simulink model "Motor_control_S32K_Final"  (R2018b)
settings: Solver=FixedStepDiscrete  StartTime=0.0  StopTime=2  RelTol=1e-3
InitFcn:
  | mbd_s32k14_consistency_checks(bdroot(gcs));
model workspace (MAT data in the model file):
  C_LST = 0.0001
  Nmax = 10000
  PP = 2
  S_LST = 0.001
undefined symbols (not defined in the file): LQFP
libraries: mbd_s32k14_ec_toolbox x13, ammclib_bam_s32k14x x9, simulink x2
Description:
  | This model is used to verify in simulation environment the correct generation
  | of PWM duty cycle commands.
  | 
  | For PWM commands generation, a special NXP library block is used.
  | The GMCLIB_SvmStd function for calculating duty-cycle ratios is widely-used
  | in the modern electric drive. This, function calculates appropriate duty-cycle
  | ratios, which are needed for generating the given stator reference voltage
  | vector using a special Space Vector Modulation technique.
  | 
  | The basic principle of Space Vector Modulation is to approximate the
  | reference stator voltage vector with an appropriate combination
  | of the switching patterns composed of basic space vectors.
  | 
  | For details, please refer to AMMCLIB User Guide, GMCLIB_SvmStd chapter.
  | 
  | For simplicity, a V/f scalar control is simulated to check the correctness of the
  | model prior of testion on the real hardware.
  | 
  | Scope of this model:
  | - demonstrate how to generate the reference signals needed for control
  | - introduce the AMMCLIB special functions for FOC transformations
  | - verify the SVM prior to testing on real hardware
settings Model: Creator=B21307  LastModifiedBy=Arjun
settings DataIOCC: ExternalInput=off  InitialState=off  SaveOutput=off  SignalLogging=off  SaveTime=off
settings OptimizationCC: DefaultParameterBehavior=Inlined  LifeSpan=inf
settings DebuggingCC: InheritedTsInSrcMsg=none  SingleTaskRateTransMsg=error  ParameterPrecisionLossMsg=none  ParameterTunabilityLossMsg=error  UnconnectedInputMsg=error  UnconnectedOutputMsg=error  UnconnectedLineMsg=error  UnknownTsInhSupMsg=error  SFExecutionAtInitializationDiag=none
settings HardwareCC: ProdBitPerPointer=32  ProdBitPerSizeT=32  ProdBitPerPtrDiffT=32  ProdLargestAtomicInteger=Long  ProdLargestAtomicFloat=Double  ProdWordSize=32  ProdHWDeviceType=ARM Compatible->ARM Cortex
settings SFSimCC: SimUseLocalCustomCode=off  MATLABDynamicMemAlloc=off
settings RTWCC: SystemTargetFile=mbd_s32k14.tlc  MakeCommand=mbd_s32k14_make_rtw COPY_MDLREF_INCLUDES=0  TemplateMakefile=mbd_s32k14.tmf  Description=Model Based Design Toolbox S32K14x Code Generation Target  RTWUseLocalCustomCode=off  IncludeHyperlinkInReport=on
settings CodeAppCC: ForceParamTrailComments=on  IgnoreCustomStorageClasses=off  OperatorAnnotations=on  SimulinkDataObjDesc=on  SFDataObjDesc=on  InsertBlockDesc=on  StateflowObjectComments=on
settings STFCustomTargetCC: TargetLangStandard=C99 (ISO)  MultiwordLength=256  CombineOutputUpdateFcns=on  ERTCustomFileBanners=on  SupportContinuousTime=off  SupportNonInlinedSFcns=off  RemoveResetFunc=on  MATLABClassNameForMDSCustomization=Simulink.SoftwareTarget.ERTCustomization  SystemTargetFile=mbd_s32k14.tlc
settings ERTTargetCC: TargetLangStandard=C99 (ISO)  ParMdlRefBuildCompliant=off  CompOptLevelCompliant=off  ConcurrentExecutionCompliant=off  ModelStepFunctionPrototypeControlCompliant=off  CPPClassGenCompliant=off  UseToolchainInfoCompliant=off  InlinedParameterPlacement=NonHierarchical  ERTCustomFileTemplate=example_file_process.tlc

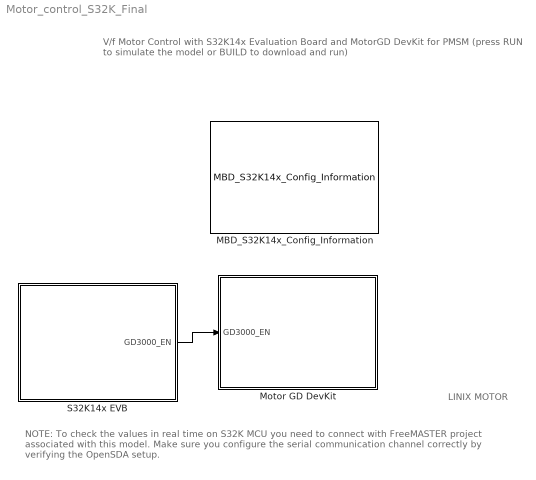
== system Motor_control_S32K_Final ==
  note: LINIX MOTOR
  note: V/f Motor Control
      | with S32K14x Evaluation Board and MotorGD DevKit for PMSM
      | (press RUN to simulate the model or BUILD to download and run)
  note: NOTE: To check the values in real time on S32K MCU you need to connect with FreeMASTER project associated with this model. Make sure you configure the serial communication channel correctly by verifying the OpenSDA setup.
  MBD_S32K14x_Config_Information : mbd_s32k14_ec_toolbox/MBD_S32K14x_Config_Information  Priority=1  disp_str=|  config_params=[]  mcu_target_name=S32K144  mcu_target_package=100-LQFP  mcu_target_sram_size=64KB  mcu_system_clock_freq=80  mcu_xtal_freq=External 8  mcu_steptick_timer=LPIT Channel 0  mcu_steptick_prio=15  ds_import_enable=on  target_compiler=GCC  target_memory=FLASH  gcc_target_compile_opts=-mcpu=cortex-m4 -mthumb -mfloat-abi=hard -mfpu=fpv4-sp-d16 -O1 -g -gstrict-dwarf  gcc_target_assemble_opts=-mcpu=cortex-m4 -mthumb -mfloat-abi=hard -mfpu=fpv4-sp-d16 -g  gcc_target_link_opts=-mcpu=cortex-m4 -mthumb -mfloat-abi=hard -mfpu=fpv4-sp-d16  gcc_target_default_lcf=on  gcc_target_user_lcf=S32K148_256_flash.ld  ghs_target_compile_opts=-cpu=cortexm4f -thumb -fpu=vfpv4_d16 -fsingle -Ogeneral -Wundef -Wimplicit-int -Wshadow -Wtrigraphs --no_commons --gnu_asm -gnu99 -gdwarf-2 -G  ghs_target_assemble_opts=-cpu=cortexm4f -fpu=vfpv4_d16  ghs_target_link_opts=-cpu=cortexm4f -thumb -fpu=vfpv4_d16  ghs_target_default_lcf=on  ghs_target_user_lcf=S32K148_256_flash.ld  iar_target_compile_opts=--cpu=Cortex-M4F --thumb --fpu=VFPv4_sp -Ol -e --debug --dlib_config normal  iar_target_assemble_opts=--cpu Cortex-M4F --thumb --fpu VFPv4_sp  iar_target_link_opts=--no_exceptions --vfe --inline  iar_target_default_lcf=on  iar_target_user_lcf=S32K148_256_flash.icf  pil_download_enable=off  rbl_download_enable=on  rbl_start_delay=5000  rbl_download_interface=OpenSDA  rbl_restart_request=off  rbl_com_port=Custom  rbl_com_port_custom=COM1  pil_download_rate=57600  pil_opensda_drive=Custom  pil_opensda_drive_custom=E  FTM_PWM_PcrCheckEnDis=on  FTM_Input_Edge_Inputs_PcrCheckEnDis=on  FTM_Dual_Edge_Inputs_PcrCheckEnDis=on  FTM_Quadrature_Inputs_PcrCheckEnDis=on  LPTMR_PcrCheckEnDis=on  PIT_PcrCheckEnDis=on  RTC_PcrCheckEnDis=on  FlexCAN_PcrCheckEnDis=on  FlexIO_PcrCheckEnDis=on  LPI2C_PcrCheckEnDis=on  LPSPI_PcrCheckEnDis=on  LPUART_PcrCheckEnDis=on  CMP_PcrCheckEnDis=on  GPIO_OutputPcrCheckEnDis=on  GPIO_InputPcrCheckEnDis=on  SBC_PcrCheckEnDis=on  AMMCLIB_PcrCheckEnDis=on  FM_PcrCheckEnDis=on  Profile_PcrCheckEnDis=on  ConfigParams_PcrCheckEnDis=on  ModelRef_PcrCheckEnDis=on  PDB0_PcrCheckEnDis=on  CSEc_PcrCheckEnDis=on  eDMA_PcrCheckEnDis=on  ADC_PcrCheckEnDis=on
      | Target : S32K144-64KB_SRAM
      | Package : 100-pin
      | System clock : 80 MHz
      | XTAL clock : External 8 MHz
      | Compiler : GCC
      | Target Type : FLASH
      | Download Code after build : (OpenSDA: D)
      | Step Tick Interrupt Priority : 15
  Motor GD DevKit : Subsystem
      mask Display: image('.\img\MotorGD.PNG');
  S32K14x EVB : Subsystem
      mask Display: image('.\img\S32K.PNG');
  wires:
  S32K14x EVB/1(GD3000_EN) -> Motor GD DevKit/1(GD3000_EN)

== system Motor_control_S32K_Final/Motor GD DevKit ==
  note: MotorGD DevKit Configuration
      |
      | PWM Commands are transformed in 3-phase Sinusoidal Voltages with Vdc amplitude
      | Enable the MC34GD3000 pre-driver to allow voltage generation on motor phases
  GD3000_EN : Inport
  GD3000_EN_IO : mbd_s32k14_ec_toolbox/GPIO Blocks/Digital_Output  gpio_pin=PTA2: [PTA2 | Port A I/O]  drive_strength=High
  GD3000_RST_IO : mbd_s32k14_ec_toolbox/GPIO Blocks/Digital_Output  gpio_pin=PTA3: [PTA3 | Port A I/O]  drive_strength=High
  ON : Constant  OutDataTypeStr=boolean
  wires:
  ON/1 -> GD3000_RST_IO/1
  GD3000_EN/1 -> GD3000_EN_IO/1

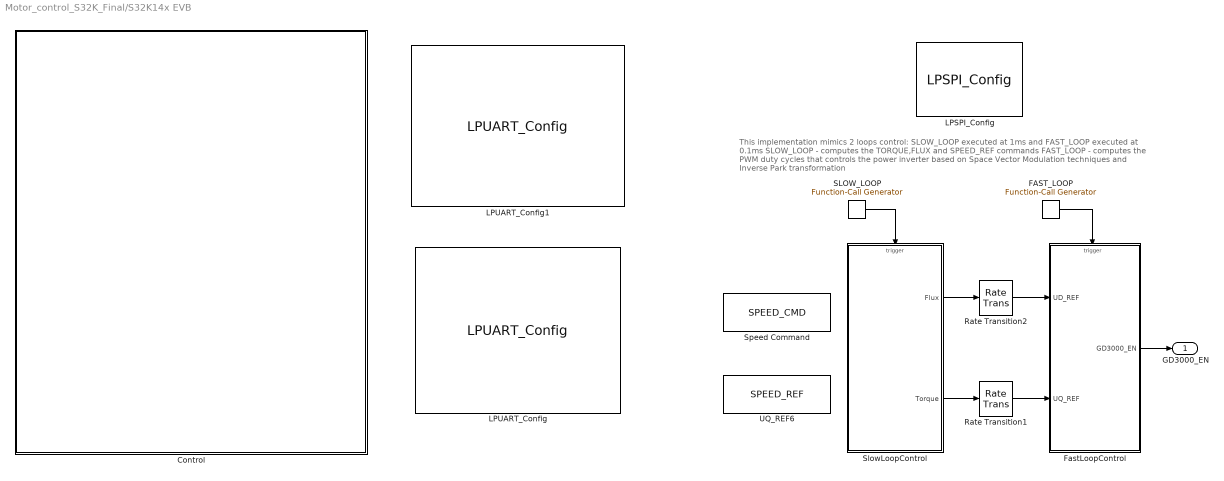
== system Motor_control_S32K_Final/S32K14x EVB ==
  note: This implementation mimics 2 loops control: SLOW_LOOP executed at 1ms and FAST_LOOP executed at 0.1ms
      | SLOW_LOOP - computes the TORQUE,FLUX and SPEED_REF  commands
      | FAST_LOOP  - computes the PWM duty cycles that controls the power inverter based on Space Vector Modulation
      |                          techniques and Inverse Park transformation
  "Control " : Subsystem
  FAST_LOOP : simulink/Ports & Subsystems/Function-Call Generator  sample_time=C_LST  numberOfIterations=1
  FastLoopControl : Subsystem
      settings: RTWFcnNameOpts=Use subsystem name
  "LPSPI_Config " : mbd_s32k14_ec_toolbox/Communication Blocks/SPI Blocks/LPSPI_Config   InstanceNumber=0  Role=Master  BaudRate=1000000  ShowAdvanced=on  sin=PTB3: [LPSPI0_SIN | LPSPI Serial Data Input]  sout=PTB4: [LPSPI0_SOUT | LPSPI Serial Data Output]  sck=PTB2: [LPSPI0_SCK | LPSPI Serial Clock I/O]  pcs0=PTB0: [LPSPI0_PCS0 | Peripheral Chip Select 0]  pcs1=PTB5: [LPSPI0_PCS1 | Peripheral Chip Select 1]  pcs2=PTE6: [LPSPI0_PCS2 | Peripheral Chip Select 2]  pcs3=PTA15: [LPSPI0_PCS3 | Peripheral Chip Select 3]  CPHA=1  CPOL=0  BitOrder=MSB first  TransferSize=8  WhichPCS=1  PCSPol=ActiveLow  ContinuousTransfer=off
  LPUART_Config : mbd_s32k14_ec_toolbox/Communication Blocks/UART Blocks/LPUART_Config  Priority=1  instance=1  baudrate=115200  databits=8  parity=None  sbns=1  bothedge=rising edge  rxinv=off  txinv=off  show_adv_opts=on  brk13=10 - 13 bit times  lbkde=10 - 13 bit times  rx=PTC6: [LPUART1_RX | Receive]  tx=PTC7: [LPUART1_TX | Transmit]  cts=PTA6: [LPUART1_CTS | Clear To Send (bar)]  rts=PTA7: [LPUART1_RTS | Request To Send]
  LPUART_Config1 : mbd_s32k14_ec_toolbox/Communication Blocks/UART Blocks/LPUART_Config  Priority=2  instance=2  baudrate=115200  databits=8  parity=None  sbns=1  bothedge=rising edge  rxinv=off  txinv=off  show_adv_opts=off  brk13=10 - 13 bit times  lbkde=10 - 13 bit times  rx=PTD6: [LPUART2_RX | Receive]  tx=PTD7: [LPUART2_TX | Transmit]  cts=PTD11: [LPUART2_CTS | Clear To Send (bar)]  rts=PTD12: [LPUART2_RTS | Request To Send]
  Rate Transition1 : RateTransition  OutPortSampleTime=C_LST
  Rate Transition2 : RateTransition  OutPortSampleTime=C_LST
  SLOW_LOOP : simulink/Ports & Subsystems/Function-Call Generator  sample_time=S_LST  numberOfIterations=1
  SlowLoopControl : Subsystem
      settings: RTWFcnNameOpts=Use subsystem name
  Speed Command : DataStoreMemory  DataStoreName=SPEED_CMD  ReadBeforeWriteMsg=warning  WriteAfterWriteMsg=warning  WriteAfterReadMsg=warning  ShowAdditionalParam=off  OutMin=-100  OutMax=200  OutDataTypeStr=single
  UQ_REF6 : DataStoreMemory  DataStoreName=SPEED_REF  ReadBeforeWriteMsg=warning  WriteAfterWriteMsg=warning  WriteAfterReadMsg=warning  ShowAdditionalParam=off  OutDataTypeStr=single
  GD3000_EN : Outport
  wires:
  SLOW_LOOP/1 -> SlowLoopControl/Trigger
  Rate Transition2/1 -> FastLoopControl/1(UD_REF)
  Rate Transition1/1 -> FastLoopControl/2(UQ_REF)
  SlowLoopControl/1(Flux) -> Rate Transition2/1
  SlowLoopControl/2(Torque) -> Rate Transition1/1
  FAST_LOOP/1 -> FastLoopControl/Trigger
  FastLoopControl/1(GD3000_EN) -> GD3000_EN/1

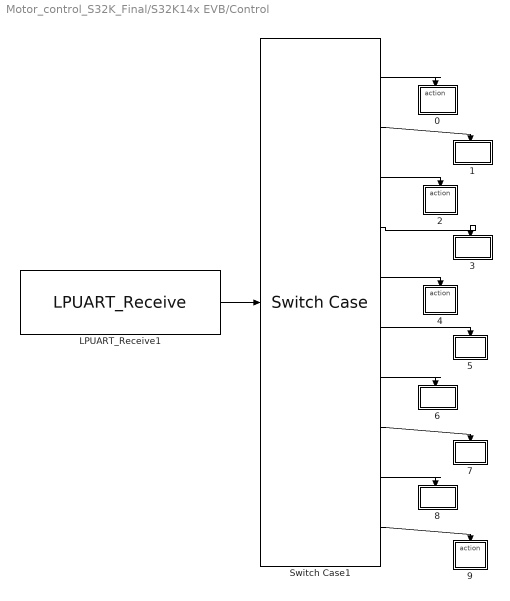
== system Motor_control_S32K_Final/S32K14x EVB/Control  ==
  0 : Subsystem  TreatAsAtomicUnit=on
  1 : Subsystem  TreatAsAtomicUnit=on
  2 : Subsystem  TreatAsAtomicUnit=on
  "3 " : Subsystem  TreatAsAtomicUnit=on
  "4 " : Subsystem  TreatAsAtomicUnit=on
  5 : Subsystem  TreatAsAtomicUnit=on
  6 : Subsystem  TreatAsAtomicUnit=on
  7 : Subsystem  TreatAsAtomicUnit=on
  "8 " : Subsystem  TreatAsAtomicUnit=on
  9 : Subsystem  TreatAsAtomicUnit=on
  LPUART_Receive1 : mbd_s32k14_ec_toolbox/Communication Blocks/UART Blocks/LPUART_Receive  Priority=1  instance=1
  Switch Case1 : SwitchCase  CaseConditions={hex2dec('030'),hex2dec('031'),hex2dec('032'),hex2dec('033'),hex2dec('034'),hex2dec('035'),hex2dec('036'),hex2dec('037'),hex2dec('038'),hex2dec('039')}  ShowDefaultCase=off
  wires:
  Switch Case1/3 -> 2/Action
  Switch Case1/8 -> 7/Action
  Switch Case1/1 -> 0/Action
  LPUART_Receive1/1 -> Switch Case1/1
  Switch Case1/6 -> 5/Action
  Switch Case1/10 -> 9/Action
  Switch Case1/9 -> "8 "/Action
  Switch Case1/5 -> "4 "/Action
  Switch Case1/4 -> "3 "/Action
  Switch Case1/2 -> 1/Action
  Switch Case1/7 -> 6/Action

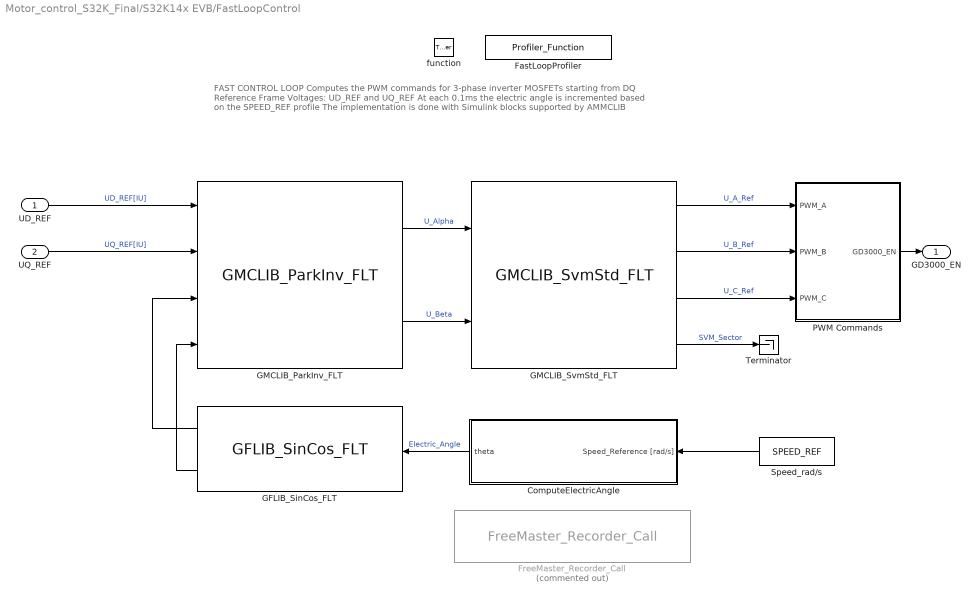
== system Motor_control_S32K_Final/S32K14x EVB/FastLoopControl ==
  note: FAST CONTROL LOOP
      |
      | Computes the PWM commands for 3-phase inverter MOSFETs starting from DQ Reference Frame Voltages: UD_REF and UQ_REF
      | At each 0.1ms the electric angle is incremented based on the SPEED_REF profile
      | The implementation is done with Simulink blocks supported by AMMCLIB
  UD_REF : Inport
  UQ_REF : Inport  Port=2
  function : TriggerPort  TriggerType=function-call  VariantControl=(inherit)
  ComputeElectricAngle : Subsystem  TreatAsAtomicUnit=on
      settings: RTWFcnNameOpts=Use subsystem name
  FastLoopProfiler : mbd_s32k14_ec_toolbox/Utility Blocks/Profiler_Function  profile_indx=0
  FreeMaster_Recorder_Call : mbd_s32k14_ec_toolbox/Utility Blocks/FreeMaster_Recorder_Call  Commented=on
  GFLIB_SinCos_FLT : ammclib_bam_s32k14x/GFLIB/bam_flt/GFLIB_SinCos_FLT
  GMCLIB_ParkInv_FLT : ammclib_bam_s32k14x/GMCLIB/bam_flt/GMCLIB_ParkInv_FLT
  GMCLIB_SvmStd_FLT : ammclib_bam_s32k14x/GMCLIB/bam_flt/GMCLIB_SvmStd_FLT
  PWM Commands : Subsystem
  Speed_rad/s : DataStoreRead  DataStoreName=SPEED_REF
  Terminator : Terminator
  GD3000_EN : Outport
  wires:
  GFLIB_SinCos_FLT/2 -> GMCLIB_ParkInv_FLT/4
  GMCLIB_ParkInv_FLT/1 -> GMCLIB_SvmStd_FLT/1  "U_Alpha"
  GMCLIB_ParkInv_FLT/2 -> GMCLIB_SvmStd_FLT/2  "U_Beta"
  GFLIB_SinCos_FLT/1 -> GMCLIB_ParkInv_FLT/3
  GMCLIB_SvmStd_FLT/2 -> PWM Commands/2(PWM_B)  "U_B_Ref"
  GMCLIB_SvmStd_FLT/3 -> PWM Commands/3(PWM_C)  "U_C_Ref"
  GMCLIB_SvmStd_FLT/4 -> Terminator/1  "SVM_Sector"
  GMCLIB_SvmStd_FLT/1 -> PWM Commands/1(PWM_A)  "U_A_Ref"
  UD_REF/1 -> GMCLIB_ParkInv_FLT/1  "UD_REF[IU]"
  UQ_REF/1 -> GMCLIB_ParkInv_FLT/2  "UQ_REF[IU]"
  ComputeElectricAngle/1(theta) -> GFLIB_SinCos_FLT/1  "Electric_Angle"
  PWM Commands/1(GD3000_EN) -> GD3000_EN/1
  Speed_rad/s/1 -> ComputeElectricAngle/1(Speed_Reference [rad/s])

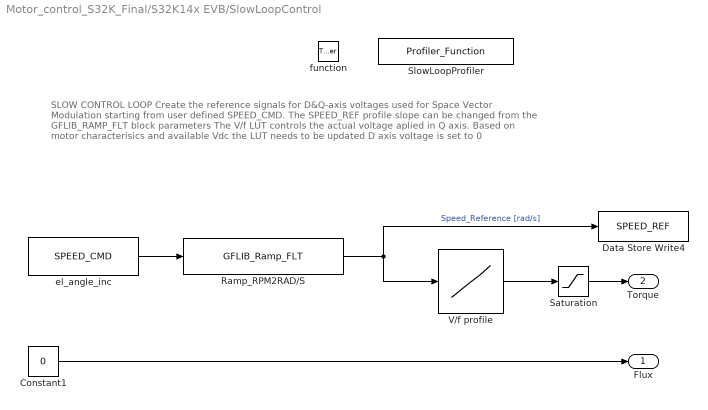
== system Motor_control_S32K_Final/S32K14x EVB/SlowLoopControl ==
  note: SLOW CONTROL LOOP
      |
      | Create the reference signals for D&Q-axis voltages used for Space Vector Modulation starting from user defined SPEED_CMD.
      | The SPEED_REF profile slope can be changed from the GFLIB_RAMP_FLT block parameters
      | The V/f LUT controls the actual voltage aplied in Q axis. Based on motor characterisics and available Vdc the LUT needs to be updated
      | D axis voltage is set to 0
  function : TriggerPort  TriggerType=function-call  VariantControl=(inherit)
  Constant1 : Constant  Value=0  OutDataTypeStr=single  SampleTime=-1
  Data Store Write4 : DataStoreWrite  DataStoreName=SPEED_REF
  Ramp_RPM2RAD/S : ammclib_bam_s32k14x/GFLIB/bam_flt/GFLIB_Ramp_FLT  fltRampUp=0.1  fltRampDown=0.1
  Saturation : Saturate  UpperLimit=0.95  LowerLimit=0
  SlowLoopProfiler : mbd_s32k14_ec_toolbox/Utility Blocks/Profiler_Function  profile_indx=1
  V/f profile : Lookup_n-D  NumberOfTableDimensions=1  BreakpointsForDimension1=[0:20.94:309.4]  Table=[0.20:0.075:0.95]  InternalRulePriority=Speed  RndMeth=Simplest  InputSameDT=on
  el_angle_inc : DataStoreRead  DataStoreName=SPEED_CMD
  Flux : Outport
  Torque : Outport  Port=2
  wires:
  Constant1/1 -> Flux/1
  V/f profile/1 -> Saturation/1
  el_angle_inc/1 -> Ramp_RPM2RAD/S/1
  Saturation/1 -> Torque/1
  Ramp_RPM2RAD/S/1 -> V/f profile/1, Data Store Write4/1  "Speed_Reference [rad/s]"

== system Motor_control_S32K_Final/S32K14x EVB/Control /0 ==
  Action Port : ActionPort  ActionType=case
  Constant : Constant  Value=0  OutDataTypeStr=single
  Data Store Write : DataStoreWrite  DataStoreName=SPEED_CMD
  wires:
  Constant/1 -> Data Store Write/1

== system Motor_control_S32K_Final/S32K14x EVB/Control /1 ==
  Action Port : ActionPort  ActionType=case
  Constant : Constant  Value=100  OutDataTypeStr=single
  Data Store Write : DataStoreWrite  DataStoreName=SPEED_CMD
  wires:
  Constant/1 -> Data Store Write/1

== system Motor_control_S32K_Final/S32K14x EVB/Control /2 ==
  Action Port : ActionPort  ActionType=case
  Constant : Constant  Value=200  OutDataTypeStr=single
  Data Store Write : DataStoreWrite  DataStoreName=SPEED_CMD
  wires:
  Constant/1 -> Data Store Write/1

== system Motor_control_S32K_Final/S32K14x EVB/Control /3  ==
  Action Port : ActionPort  ActionType=case
  Constant : Constant  Value=300  OutDataTypeStr=single
  Data Store Write : DataStoreWrite  DataStoreName=SPEED_CMD
  wires:
  Constant/1 -> Data Store Write/1

== system Motor_control_S32K_Final/S32K14x EVB/Control /4  ==
  Action Port : ActionPort  ActionType=case
  Constant : Constant  Value=400  OutDataTypeStr=single
  Data Store Write : DataStoreWrite  DataStoreName=SPEED_CMD
  wires:
  Constant/1 -> Data Store Write/1

== system Motor_control_S32K_Final/S32K14x EVB/Control /5 ==
  Action Port : ActionPort  ActionType=case
  Constant : Constant  Value=500  OutDataTypeStr=single
  Data Store Write : DataStoreWrite  DataStoreName=SPEED_CMD
  wires:
  Constant/1 -> Data Store Write/1

== system Motor_control_S32K_Final/S32K14x EVB/Control /6 ==
  Action Port : ActionPort  ActionType=case
  Constant : Constant  Value=600  OutDataTypeStr=single
  Data Store Write : DataStoreWrite  DataStoreName=SPEED_CMD
  wires:
  Constant/1 -> Data Store Write/1

== system Motor_control_S32K_Final/S32K14x EVB/Control /7 ==
  Action Port : ActionPort  ActionType=case
  Constant : Constant  Value=800  OutDataTypeStr=single
  Data Store Write1 : DataStoreWrite  DataStoreName=SPEED_REF
  wires:
  Constant/1 -> Data Store Write1/1

== system Motor_control_S32K_Final/S32K14x EVB/Control /8  ==
  Action Port : ActionPort  ActionType=case
  Constant : Constant  Value=2100  OutDataTypeStr=single
  Data Store Write : DataStoreWrite  DataStoreName=SPEED_REF
  wires:
  Constant/1 -> Data Store Write/1

== system Motor_control_S32K_Final/S32K14x EVB/Control /9 ==
  Action Port : ActionPort  ActionType=case
  Constant : Constant  Value=4000  OutDataTypeStr=single
  Data Store Write1 : DataStoreWrite  DataStoreName=SPEED_REF
  wires:
  Constant/1 -> Data Store Write1/1

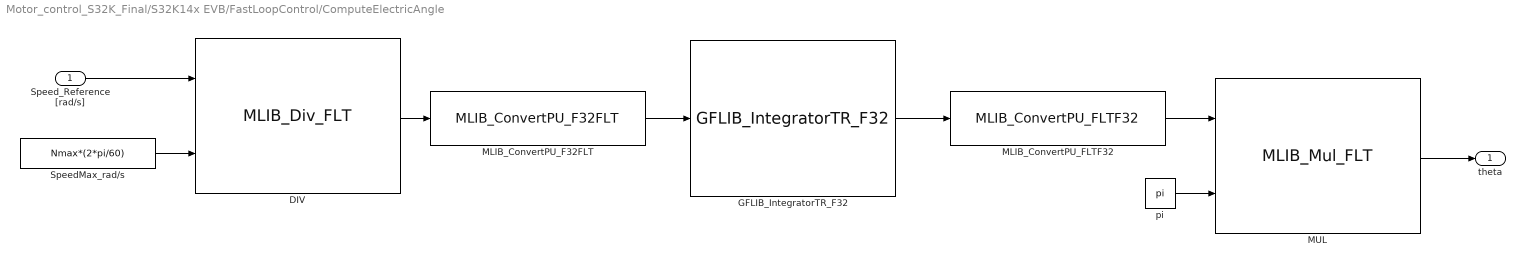
== system Motor_control_S32K_Final/S32K14x EVB/FastLoopControl/ComputeElectricAngle ==
  Speed_Reference [rad/s] : Inport
  DIV : ammclib_bam_s32k14x/MLIB/bam_flt/MLIB_Div_FLT
  GFLIB_IntegratorTR_F32 : ammclib_bam_s32k14x/GFLIB/bam_f32/GFLIB_IntegratorTR_F32  f32C1=(2*pi/60)*PP*Nmax*(C_LST/2/pi)*(2^31)  u16NShift=0
  MLIB_ConvertPU_F32FLT : ammclib_bam_s32k14x/MLIB/bam_f32/MLIB_ConvertPU_F32FLT
  MLIB_ConvertPU_FLTF32 : ammclib_bam_s32k14x/MLIB/bam_flt/MLIB_ConvertPU_FLTF32
  MUL : ammclib_bam_s32k14x/MLIB/bam_flt/MLIB_Mul_FLT
  SpeedMax_rad/s : Constant  Value=Nmax*(2*pi/60)  OutDataTypeStr=Inherit: Inherit via back propagation
  pi : Constant  Value=pi  OutDataTypeStr=Inherit: Inherit via back propagation
  theta : Outport  OutDataTypeStr=single
  wires:
  pi/1 -> MUL/2
  GFLIB_IntegratorTR_F32/1 -> MLIB_ConvertPU_FLTF32/1
  MLIB_ConvertPU_F32FLT/1 -> GFLIB_IntegratorTR_F32/1
  MLIB_ConvertPU_FLTF32/1 -> MUL/1
  MUL/1 -> theta/1
  Speed_Reference [rad/s]/1 -> DIV/1
  DIV/1 -> MLIB_ConvertPU_F32FLT/1
  SpeedMax_rad/s/1 -> DIV/2

== system Motor_control_S32K_Final/S32K14x EVB/FastLoopControl/PWM Commands ==
  PWM_A : Inport
  PWM_B : Inport  Port=2
  PWM_C : Inport  Port=3
  Control_Logic : Subsystem
  Demux : Demux  Outputs=6
  FTM_PWM_Config : mbd_s32k14_ec_toolbox/Motor Control Blocks/FTM Blocks/FTM_PWM_Config  ftmModule=3  ftmMode=Center-Aligned PWM  ftmSourceClock=80 MHz  chan0En=on  chan0Type=Independent  chan2En=on  chan2Type=Independent  chan4En=on  chan4Type=Independent  chan6En=off  chan6Type=Independent  ftmPwmUnits=Hz  outFrequency=20000  ftmPeriod=4000  ftmPrescaler=Divide by 1  deadtimeUnits=Ticks  deadtimeNs=0  deadtimeTicks=0  deadtimePrescaler=Divide by 1  dutyCycleCh0=0  dutyCycleCh1=0  dutyCycleCh2=0  dutyCycleCh3=0  dutyCycleCh4=0  dutyCycleCh5=0  dutyCycleCh6=0.25  dutyCycleCh7=0.25  dutyCycleSim=off  startAfterInit=off  showAdvOpt=on  pinFtmCh0=PTB8: [FTM3_CH0 | FTM Channel]  pinFtmCh1=PTB9: [FTM3_CH1 | FTM Channel]  pinPolCh0=Active Low  pinPolCh1=Main duplicated  outputLevel0=Low-true pulses  outputLevel1=High-true pulses  pinFtmCh2=PTB10: [FTM3_CH2 | FTM Channel]  pinFtmCh3=PTB11: [FTM3_CH3 | FTM Channel]  pinPolCh2=Active Low  pinPolCh3=Main duplicated  outputLevel2=Low-true pulses  outputLevel3=High-true pulses  pinFtmCh4=PTC10: [FTM3_CH4 | FTM Channel]  pinFtmCh5=PTC11: [FTM3_CH5 | FTM Channel]  pinPolCh4=Active Low  pinPolCh5=Main duplicated  outputLevel4=Low-true pulses  outputLevel5=High-true pulses  pinFtmCh6=PTC12: [FTM3_CH6 | FTM Channel]  pinFtmCh7=None  pinPolCh6=Active Low  pinPolCh7=Main duplicated  outputLevel6=High-true pulses  outputLevel7=High-true pulses  initTrigger=off  chTrigger0=off  chTrigger1=off  chTrigger2=off  chTrigger3=off  chTrigger4=off  chTrigger5=off  chTrigger6=off  chTrigger7=off  mcuTargetUpdate=on  pwmSyncTrg=Software trigger  pwmSyncHwRouting=TRGMUX_FTM7  pwmSyncTrg0=off  pwmSyncTrg1=off  pwmSyncTrg2=off  pwmSyncAutoClear=on  pwmSyncMinLoad=on  pwmSyncMaxLoad=on  pwmSyncInvert=System Clock  pwmSyncOutControl=System Clock  pwmSyncOutMask=System Clock  pwmSyncCounterInitial=System Clock  pwmSyncPoints=Update now  reloadEnable=off  reloadPriority=15  reloadHalfCycle=off  reloadHCR=0  reloadFrequency=0  chnMatch0=off  chnMatch1=off  chnMatch2=off  chnMatch3=off  chnMatch4=off  chnMatch5=off  chnMatch6=off  chnMatch7=off  pwmFaultProtection=off  pwmFaultInterrupt=off  pwmFaultClearing=Fault control disabled  pwmFaultPinState=Safe Value  pwmFaultFilterValue=0  pwmFaultPriority=15  fault_disen_0=off  fault_filter_0=off  fault_polarity_0=Active High  fault_disen_1=off  fault_filter_1=off  fault_polarity_1=Active high  fault_disen_2=off  fault_filter_2=off  fault_polarity_2=Active high  fault_disen_3=off  fault_filter_3=off  fault_polarity_3=Active high  fault_pin_0=None  fault_pin_1=None  fault_pin_2=None  fault_pin_3=None
  Mux : Mux  Inputs=6
  GD3000_EN : Outport
  wires:
  Mux/1 -> Control_Logic/1(PWM)
  Control_Logic/1("PWM ") -> Demux/1
  Control_Logic/2(GD3000_EN) -> GD3000_EN/1
  Demux/2 -> FTM_PWM_Config/2  "PA_LS"
  Demux/1 -> FTM_PWM_Config/1  "PA_HS"
  Demux/3 -> FTM_PWM_Config/3  "PB_HS"
  Demux/4 -> FTM_PWM_Config/4  "PB_LS"
  Demux/5 -> FTM_PWM_Config/5  "PC_HS"
  Demux/6 -> FTM_PWM_Config/6  "PC_LS"
  PWM_A/1 -> Mux/2, Mux/1  "PWM_A"
  PWM_B/1 -> Mux/3, Mux/4  "PWM_B"
  PWM_C/1 -> Mux/6, Mux/5  "PWM_C"

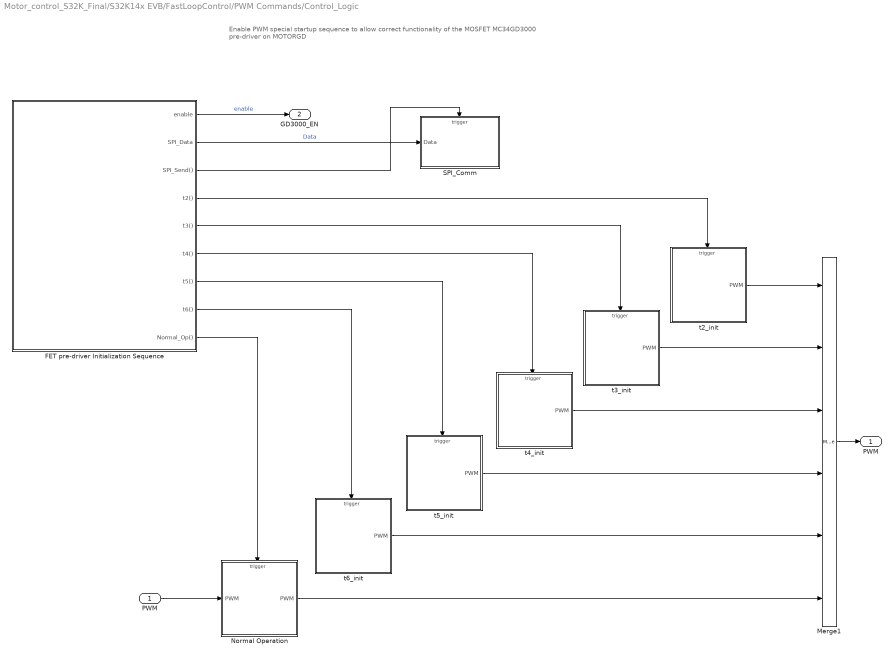
== system Motor_control_S32K_Final/S32K14x EVB/FastLoopControl/PWM Commands/Control_Logic ==
  note: Enable PWM special startup sequence to allow correct functionality of the MOSFET MC34GD3000 pre-driver on MOTORGD
  PWM : Inport
  FET pre-driver Initialization Sequence : Stateflow chart  TreatAsAtomicUnit=on
  Merge1 : Merge  Inputs=6
  Normal Operation : Subsystem  TreatAsAtomicUnit=on
  SPI_Comm : Subsystem
  t2_init : Subsystem  TreatAsAtomicUnit=on
  t3_init : Subsystem  TreatAsAtomicUnit=on
  t4_init : Subsystem  TreatAsAtomicUnit=on
  t5_init : Subsystem  TreatAsAtomicUnit=on
  t6_init : Subsystem  TreatAsAtomicUnit=on
  "PWM " : Outport
  GD3000_EN : Outport  Port=2
  wires:
  FET pre-driver Initialization Sequence/8(t6()) -> t6_init/Trigger
  FET pre-driver Initialization Sequence/7(t5()) -> t5_init/Trigger
  PWM/1 -> Normal Operation/1("PWM ")
  FET pre-driver Initialization Sequence/1(enable) -> GD3000_EN/1  "enable"
  FET pre-driver Initialization Sequence/9(Normal_Op()) -> Normal Operation/Trigger
  FET pre-driver Initialization Sequence/6(t4()) -> t4_init/Trigger
  FET pre-driver Initialization Sequence/5(t3()) -> t3_init/Trigger
  FET pre-driver Initialization Sequence/4(t2()) -> t2_init/Trigger
  Normal Operation/1(PWM) -> Merge1/6
  Merge1/1 -> "PWM "/1
  t2_init/1(PWM) -> Merge1/1
  t3_init/1(PWM) -> Merge1/2
  t4_init/1(PWM) -> Merge1/3
  t5_init/1(PWM) -> Merge1/4
  t6_init/1(PWM) -> Merge1/5
  FET pre-driver Initialization Sequence/2(SPI_Data) -> SPI_Comm/1(Data)  "Data"
  FET pre-driver Initialization Sequence/3(SPI_Send()) -> SPI_Comm/Trigger

== system Motor_control_S32K_Final/S32K14x EVB/FastLoopControl/PWM Commands/Control_Logic/Normal Operation ==
  "PWM " : Inport  OutDataTypeStr=single
  function : TriggerPort  TriggerType=function-call  VariantControl=(inherit)
  PWM : Outport  InitialOutput=0
  wires:
  "PWM "/1 -> PWM/1

== system Motor_control_S32K_Final/S32K14x EVB/FastLoopControl/PWM Commands/Control_Logic/SPI_Comm ==
  Data : Inport
  function : TriggerPort  TriggerType=function-call  VariantControl=(inherit)
  LPSPI_Master_Transfer : mbd_s32k14_ec_toolbox/Communication Blocks/SPI Blocks/LPSPI_Master_Transfer  instance=0  xfermode=Non blocking  timeout=50  spi_upd=on
  Terminator : Terminator
  wires:
  Data/1 -> LPSPI_Master_Transfer/1
  LPSPI_Master_Transfer/1 -> Terminator/1

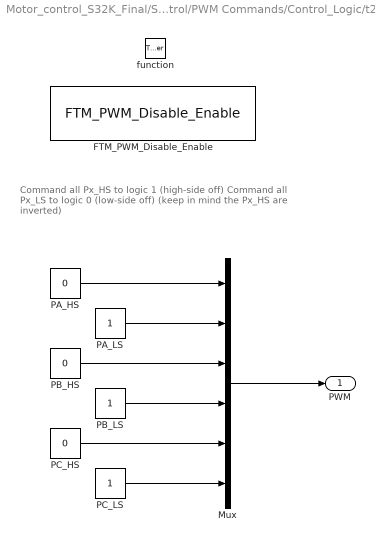
== system Motor_control_S32K_Final/S32K14x EVB/FastLoopControl/PWM Commands/Control_Logic/t2_init ==
  note: Command all Px_HS to logic 1 (high-side off)
      | Command all Px_LS to logic 0 (low-side off)
      | (keep in mind the Px_HS are inverted)
  function : TriggerPort  TriggerType=function-call  VariantControl=(inherit)
  FTM_PWM_Disable_Enable : mbd_s32k14_ec_toolbox/Motor Control Blocks/FTM Blocks/FTM_PWM_Disable_Enable  Priority=1  module=3  action=Enable
  Mux : Mux  Inputs=6
  PA_HS : Constant  Value=0  OutDataTypeStr=single  SampleTime=-1
  PA_LS : Constant  OutDataTypeStr=single  SampleTime=-1
  PB_HS : Constant  Value=0  OutDataTypeStr=single  SampleTime=-1
  PB_LS : Constant  OutDataTypeStr=single  SampleTime=-1
  PC_HS : Constant  Value=0  OutDataTypeStr=single  SampleTime=-1
  PC_LS : Constant  OutDataTypeStr=single  SampleTime=-1
  PWM : Outport  OutDataTypeStr=single  InitialOutput=0
  wires:
  PA_HS/1 -> Mux/1
  Mux/1 -> PWM/1
  PA_LS/1 -> Mux/2
  PB_HS/1 -> Mux/3
  PB_LS/1 -> Mux/4
  PC_HS/1 -> Mux/5
  PC_LS/1 -> Mux/6

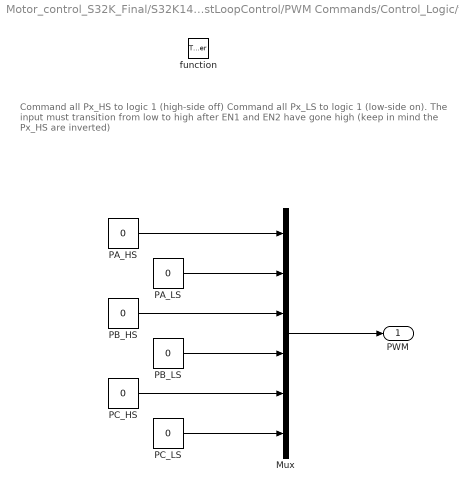
== system Motor_control_S32K_Final/S32K14x EVB/FastLoopControl/PWM Commands/Control_Logic/t3_init ==
  note: Command all Px_HS to logic 1 (high-side off)
      | Command all Px_LS to logic 1 (low-side on). The input must transition from low to high after EN1 and EN2 have gone high
      | (keep in mind the Px_HS are inverted)
  function : TriggerPort  TriggerType=function-call  VariantControl=(inherit)
  Mux : Mux  Inputs=6
  PA_HS : Constant  Value=0  OutDataTypeStr=single  SampleTime=-1
  PA_LS : Constant  Value=0  OutDataTypeStr=single  SampleTime=-1
  PB_HS : Constant  Value=0  OutDataTypeStr=single  SampleTime=-1
  PB_LS : Constant  Value=0  OutDataTypeStr=single  SampleTime=-1
  PC_HS : Constant  Value=0  OutDataTypeStr=single  SampleTime=-1
  PC_LS : Constant  Value=0  OutDataTypeStr=single  SampleTime=-1
  PWM : Outport  OutDataTypeStr=single  InitialOutput=0
  wires:
  PC_LS/1 -> Mux/6
  PC_HS/1 -> Mux/5
  PB_LS/1 -> Mux/4
  PB_HS/1 -> Mux/3
  PA_LS/1 -> Mux/2
  Mux/1 -> PWM/1
  PA_HS/1 -> Mux/1

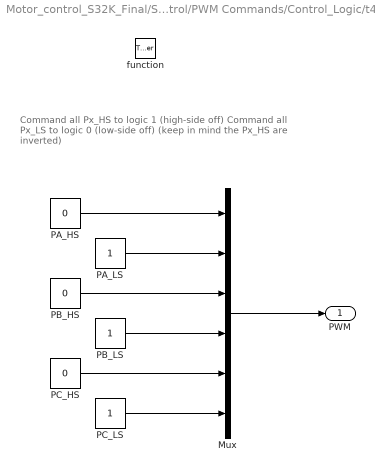
== system Motor_control_S32K_Final/S32K14x EVB/FastLoopControl/PWM Commands/Control_Logic/t4_init ==
  note: Command all Px_HS to logic 1 (high-side off)
      | Command all Px_LS to logic 0 (low-side off)
      | (keep in mind the Px_HS are inverted)
  function : TriggerPort  TriggerType=function-call  VariantControl=(inherit)
  Mux : Mux  Inputs=6
  PA_HS : Constant  Value=0  OutDataTypeStr=single  SampleTime=-1
  PA_LS : Constant  OutDataTypeStr=single  SampleTime=-1
  PB_HS : Constant  Value=0  OutDataTypeStr=single  SampleTime=-1
  PB_LS : Constant  OutDataTypeStr=single  SampleTime=-1
  PC_HS : Constant  Value=0  OutDataTypeStr=single  SampleTime=-1
  PC_LS : Constant  OutDataTypeStr=single  SampleTime=-1
  PWM : Outport  OutDataTypeStr=single  InitialOutput=0
  wires:
  PC_LS/1 -> Mux/6
  PC_HS/1 -> Mux/5
  PB_LS/1 -> Mux/4
  PB_HS/1 -> Mux/3
  PA_LS/1 -> Mux/2
  Mux/1 -> PWM/1
  PA_HS/1 -> Mux/1

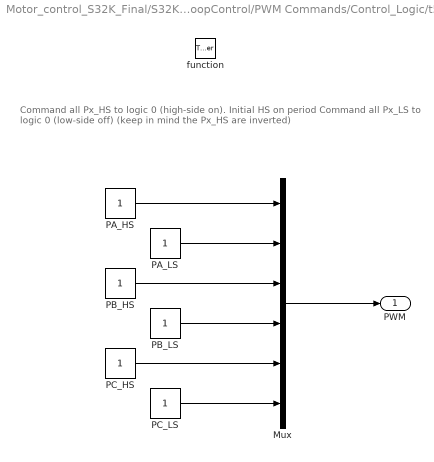
== system Motor_control_S32K_Final/S32K14x EVB/FastLoopControl/PWM Commands/Control_Logic/t5_init ==
  note: Command all Px_HS to logic 0 (high-side on). Initial HS on period
      | Command all Px_LS to logic 0 (low-side off)
      | (keep in mind the Px_HS are inverted)
  function : TriggerPort  TriggerType=function-call  VariantControl=(inherit)
  Mux : Mux  Inputs=6
  PA_HS : Constant  OutDataTypeStr=single  SampleTime=-1
  PA_LS : Constant  OutDataTypeStr=single  SampleTime=-1
  PB_HS : Constant  OutDataTypeStr=single  SampleTime=-1
  PB_LS : Constant  OutDataTypeStr=single  SampleTime=-1
  PC_HS : Constant  OutDataTypeStr=single  SampleTime=-1
  PC_LS : Constant  OutDataTypeStr=single  SampleTime=-1
  PWM : Outport  OutDataTypeStr=single  InitialOutput=0
  wires:
  PA_HS/1 -> Mux/1
  Mux/1 -> PWM/1
  PA_LS/1 -> Mux/2
  PB_HS/1 -> Mux/3
  PB_LS/1 -> Mux/4
  PC_HS/1 -> Mux/5
  PC_LS/1 -> Mux/6

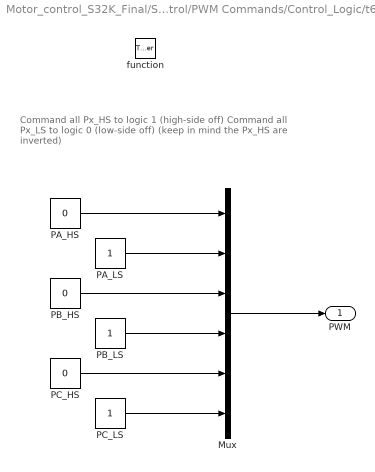
== system Motor_control_S32K_Final/S32K14x EVB/FastLoopControl/PWM Commands/Control_Logic/t6_init ==
  note: Command all Px_HS to logic 1 (high-side off)
      | Command all Px_LS to logic 0 (low-side off)
      | (keep in mind the Px_HS are inverted)
  function : TriggerPort  TriggerType=function-call  VariantControl=(inherit)
  Mux : Mux  Inputs=6
  PA_HS : Constant  Value=0  OutDataTypeStr=single  SampleTime=-1
  PA_LS : Constant  OutDataTypeStr=single  SampleTime=-1
  PB_HS : Constant  Value=0  OutDataTypeStr=single  SampleTime=-1
  PB_LS : Constant  OutDataTypeStr=single  SampleTime=-1
  PC_HS : Constant  Value=0  OutDataTypeStr=single  SampleTime=-1
  PC_LS : Constant  OutDataTypeStr=single  SampleTime=-1
  PWM : Outport  OutDataTypeStr=single  InitialOutput=0
  wires:
  PA_HS/1 -> Mux/1
  Mux/1 -> PWM/1
  PA_LS/1 -> Mux/2
  PB_HS/1 -> Mux/3
  PB_LS/1 -> Mux/4
  PC_HS/1 -> Mux/5
  PC_LS/1 -> Mux/6

== stateflow chart Motor_control_S32K_Final/S32K14x EVB/FastLoopControl/PWM Commands/Control_Logic/FET pre-driver Initialization Sequence ==
  settings: sampleTime=0.500
  note: Assumption: @80MHz index++ instruction will take ~100ns
  state A
    A -> A [order 1] : {index++;}
  state B
  state C
  state C1
  state C2
  state C3
  state C4
  state D
    D -> D [order 1] : {index++;}
  state E
    E -> E [order 1] : {index++;}
  state F
    F -> F [order 1] : {index++;}
  state G
    G -> G [order 1] : {index++;}
  state H
    H -> H [order 1] : {index++;}
  state END
  (default) -> A : {enable=0;
      | index = 0;}
  A -> B [order 1] : /*MASK0*/
      | [index > 20]
      | {SPI_Data = 0x20;
      | SPI_Send;
      | index = 0;}
  B -> C : /*MASK1*/
      | {SPI_Data = 0x30;
      | SPI_Send;}
  C -> C1 : /*CLINT0*/
      | {SPI_Data = 0x6F;
      | SPI_Send;}
  C1 -> C2 : /*CLINT1*/
      | {SPI_Data = 0x7F;
      | SPI_Send;}
  C2 -> C3 : /*DEADTIME CMD*/
      | {SPI_Data = 0x81;
      | SPI_Send;}
  C3 -> C4 : /*DEADTIME CALIBRATION PULSE*/
      | /*Set a 500ns deadtime based on the SPI CS 1Mbs Clock*/
      | {SPI_Data = 0x00;
      | SPI_Send;}
  C4 -> D : /*Mode*/
      | {SPI_Data  = 0x49;
      | SPI_Send;}
  D -> E [order 1] : /*Enable GD3000*/
      | [index > 20]
      | {SPI_Data = 0x00;
      | enable=1; t2}
  E -> F [order 1] : /*Wait 280ns for EN1 & EN2 propagation delay*/
      | [index > 3]
      | {t3;index=0;}
  F -> G [order 1] : /*Wait for the bootstrap capacitors to charge 1us*/
      | [index > 10]
      | {t4;index=0;}
  G -> H [order 1] : /*Initial HS on period*/
      | [index > 1]{t5; index = 0;}
  H -> END [order 1] : /*HS off for normal operation*/
      | [index >1]{t6;index = 0;}
  END -> END : {Normal_Op;}
  data: enable output boolean; SPI_Data output uint8; index local double
  events: SPI_Send output FUNCTION_CALL_EVENT; t2 output FUNCTION_CALL_EVENT; t3 output FUNCTION_CALL_EVENT; t4 output FUNCTION_CALL_EVENT; t5 output FUNCTION_CALL_EVENT; t6 output FUNCTION_CALL_EVENT; Normal_Op output FUNCTION_CALL_EVENT
